simulink model "EulerKinematics"  (Simulink 10.3)
settings: Solver=ode5  StartTime=0.0  StopTime=100  FixedStep=0.01  RelTol=1e-3
settings Model: Creator=PC  LastModifiedBy=PC
settings SolverCC: AlgebraicLoopSolver=Auto
settings DataIOCC: SaveFormat=Dataset  SignalLoggingSaveFormat=Dataset  ReturnWorkspaceOutputs=on
settings OptimizationCC: ExpressionDepthLimit=128  LifeSpan=auto
settings DebuggingCC: UnderspecifiedInitializationDetection=Simplified  MergeDetectMultiDrivingBlocksExec=error  FcnCallInpInsideContextMsg=error  StateNameClashWarn=none  SFUnexpectedBacktrackingDiag=error  SFNoUnconditionalDefaultTransitionDiag=error  SFExecutionAtInitializationDiag=warning  SFMachineParentedDataDiag=error  ArithmeticOperatorsInVariantConditions=error
settings HardwareCC: ProdBitPerPointer=64  ProdBitPerSizeT=64  ProdBitPerPtrDiffT=64  ProdLargestAtomicFloat=Float  ProdIntDivRoundTo=Zero  ProdEndianess=LittleEndian  ProdWordSize=64  ProdHWDeviceType=Intel->x86-64 (Windows64)
settings ModelReferenceCC: PropagateSignalLabelsOutOfModel=on
settings SFSimCC: SimUseLocalCustomCode=on  CustomCodeUndefinedFunction=FilterOut
settings RTWCC: RTWUseLocalCustomCode=on
settings CodeAppCC: StateflowObjectComments=off
settings GRTTargetCC: TargetLangStandard=C99 (ISO)  CombineOutputUpdateFcns=on  GRTInterface=off
settings ConfigComp: CovMetricSettings=dwe  CovSaveCumulativeToWorkspaceVar=off  CovSaveSingleToWorkspaceVar=off  CovExternalEMLEnable=on

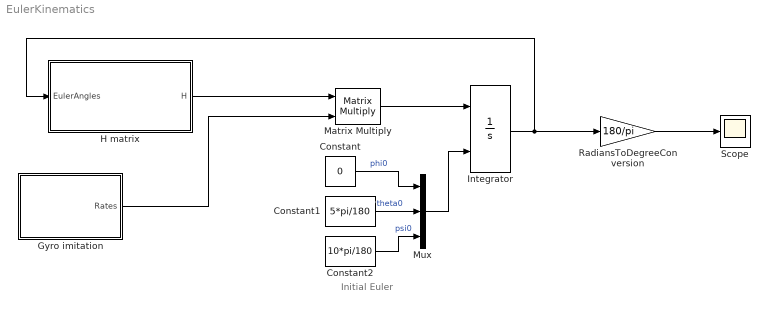
== system EulerKinematics ==
  note: Initial Euler
  Constant : Constant  Value=0
  Constant1 : Constant  Value=5*pi/180
  Constant2 : Constant  Value=10*pi/180
  Gyro imitation : Subsystem
  H matrix : MATLAB Function  TreatAsAtomicUnit=on
  Integrator : Integrator  InitialConditionSource=external
  Matrix Multiply : Product  Multiplication=Matrix(*)
  Mux : Mux  Inputs=3
  RadiansToDegreeConversion : Gain  Gain=180/pi
  Scope : Scope
  wires:
  H matrix/1(H) -> Matrix Multiply/1
  Matrix Multiply/1 -> Integrator/1
  Gyro imitation/1(Rates) -> Matrix Multiply/2
  Integrator/1 -> RadiansToDegreeConversion/1, H matrix/1(EulerAngles)
  Mux/1 -> Integrator/2
  Constant/1 -> Mux/1  "phi0"
  Constant1/1 -> Mux/2  "theta0"
  Constant2/1 -> Mux/3  "psi0"
  RadiansToDegreeConversion/1 -> Scope/1

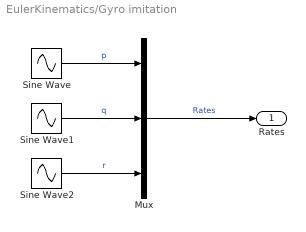
== system EulerKinematics/Gyro imitation ==
  Mux : Mux  Inputs=3
  Sine Wave : Sin  Amplitude=10*pi/180  Frequency=5*pi/180  SampleTime=0
  Sine Wave1 : Sin  Amplitude=5*pi/180  Frequency=5*pi/180  SampleTime=0
  Sine Wave2 : Sin  Amplitude=1*pi/180  Frequency=5*pi/180  SampleTime=0
  Rates : Outport
  wires:
  Mux/1 -> Rates/1  "Rates"
  Sine Wave/1 -> Mux/1  "p"
  Sine Wave1/1 -> Mux/2  "q"
  Sine Wave2/1 -> Mux/3  "r"

== matlab function H matrix ==
  data: EulerAngles input double; H output double
function H = fcn(EulerAngles)

phi = EulerAngles(1);
theta = EulerAngles(2);
psi = EulerAngles(3); 


H = [[1 tan(theta)*sin(phi) tan(theta)*cos(phi)];
    [0 cos(phi) -sin(phi)];
    [0 sin(phi)/cos(theta) cos(phi)/cos(theta)]];
